simulink model "simulacion"  (R2021a)
settings: Solver=VariableStepAuto  StartTime=0.0  StopTime=1000  RelTol=1e-3
values from neighbouring files (symbols this model uses):
  h0 = 0.45    [act4.mat]
  u0 = 0.5    [act4.mat]
libraries: cstblocks x3
settings Model: Creator=franc  LastModifiedBy=franc

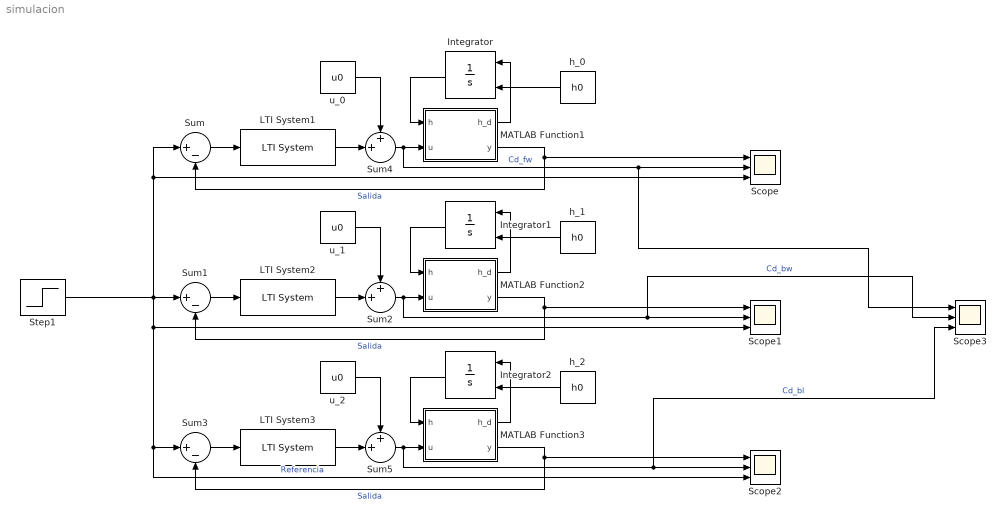
== system simulacion ==
  Integrator : Integrator  InitialConditionSource=external
  Integrator1 : Integrator  InitialConditionSource=external
  Integrator2 : Integrator  InitialConditionSource=external
  LTI System1 : cstblocks/LTI System  sys=Cd_fw  IC=[]
  LTI System2 : cstblocks/LTI System  sys=Cd_bw  IC=[]
  LTI System3 : cstblocks/LTI System  sys=Cd_bl  IC=[]
  MATLAB Function1 : MATLAB Function  TreatAsAtomicUnit=on
  MATLAB Function2 : MATLAB Function  TreatAsAtomicUnit=on
  MATLAB Function3 : MATLAB Function  TreatAsAtomicUnit=on
  Scope{,1..3} (4 alike) : Scope  NumInputPorts=3
  Step1 : Step  Time=50  Before=0.45  After=0.55  SampleTime=0
  Sum : Sum  Inputs=|+-
  Sum1 : Sum  Inputs=|+-
  Sum2 : Sum  Inputs=++|
  Sum3 : Sum  Inputs=|+-
  Sum4 : Sum  Inputs=++|
  Sum5 : Sum  Inputs=++|
  h_0 : Constant  Value=h0
  h_1 : Constant  Value=h0
  h_2 : Constant  Value=h0
  u_0 : Constant  Value=u0
  u_1 : Constant  Value=u0
  u_2 : Constant  Value=u0
  wires:
  u_0/1 -> Sum4/1
  Integrator/1 -> MATLAB Function1/1(h)
  Sum/1 -> LTI System1/1
  MATLAB Function1/1(h_d) -> Integrator/1
  MATLAB Function1/2(y) -> Scope/1, Sum/2  "Salida"
  LTI System1/1 -> Sum4/2
  h_0/1 -> Integrator/2
  Sum4/1 -> Scope3/1, Scope/2, MATLAB Function1/2(u)  "Cd_fw"
  Sum2/1 -> Scope3/2, Scope1/2, MATLAB Function2/2(u)  "Cd_bw"
  LTI System2/1 -> Sum2/2
  h_1/1 -> Integrator1/2
  u_1/1 -> Sum2/1
  Integrator1/1 -> MATLAB Function2/1(h)
  Sum1/1 -> LTI System2/1
  MATLAB Function2/2(y) -> Scope1/1, Sum1/2  "Salida"
  MATLAB Function2/1(h_d) -> Integrator1/1
  Sum5/1 -> Scope3/3, Scope2/2, MATLAB Function3/2(u)  "Cd_bl"
  LTI System3/1 -> Sum5/2
  h_2/1 -> Integrator2/2
  u_2/1 -> Sum5/1
  Integrator2/1 -> MATLAB Function3/1(h)
  Sum3/1 -> LTI System3/1
  MATLAB Function3/2(y) -> Scope2/1, Sum3/2  "Salida"
  Step1/1 -> Scope2/3, Sum3/1, Scope1/3, Sum/1, Scope/3, Sum1/1  "Referencia"
  MATLAB Function3/1(h_d) -> Integrator2/1

== matlab function simulacion/MATLAB Function1 ==
  data: h input; h_d output; u input; y output
function [h_d, y] = fcn(h, u)
    g = 9.8;        %En metros sobre segundo cuadrado
    H = 0.9;        %En metros
    L_s = 0.4;      %En metros
    L_i = 0.1;      %En metros
    d2 = 10.65e-3;
    Q_i = 0.0001333; %Metros cubicos por segundo 
    A_o = pi * (d2 / 2)^2;

    h_d = (H^2 * (Q_i - A_o * sqrt(2*g*h)*u))/(h^2*(L_s-L_i)^2 + 2*h*L_i*(L_s-L_i)*H+L_i^2*H^2);
    y = h;
end

== matlab function simulacion/MATLAB Function2 ==
  data: h input; h_d output; u input; y output
function [h_d, y] = fcn(h, u)
    g = 9.8;        %En metros sobre segundo cuadrado
    H = 0.9;        %En metros
    L_s = 0.4;      %En metros
    L_i = 0.1;      %En metros
    d2 = 10.65e-3;
    Q_i = 0.0001333; %Metros cubicos por segundo 
    A_o = pi * (d2 / 2)^2;

    h_d = (H^2 * (Q_i - A_o * sqrt(2*g*h)*u))/(h^2*(L_s-L_i)^2 + 2*h*L_i*(L_s-L_i)*H+L_i^2*H^2);
    y = h;
end

== matlab function simulacion/MATLAB Function3 ==
  data: h input; h_d output; u input; y output
function [h_d, y] = fcn(h, u)
    g = 9.8;        %En metros sobre segundo cuadrado
    H = 0.9;        %En metros
    L_s = 0.4;      %En metros
    L_i = 0.1;      %En metros
    d2 = 10.65e-3;
    Q_i = 0.0001333; %Metros cubicos por segundo 
    A_o = pi * (d2 / 2)^2;

    h_d = (H^2 * (Q_i - A_o * sqrt(2*g*h)*u))/(h^2*(L_s-L_i)^2 + 2*h*L_i*(L_s-L_i)*H+L_i^2*H^2);
    y = h;
end
